simulink library "HILeg_Lib"  (R2014a)
settings: Solver=ode45  StartTime=0.0  StopTime=10.0  RelTol=1e-3
undefined symbols (not defined in the file): k_gx, k_gy, mu_slide, mu_stick, sgn, t_friction, v_gx_max, v_gy_max, vLimit
libraries: nesl_utility x7, simulink x5, sm_lib x3, simulink_extras x1
settings Model: Creator=rshum  LastModifiedBy=rshum

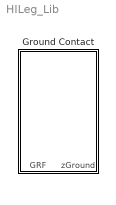
== system HILeg_Lib ==
  Ground Contact : Subsystem  SystemSampleTime=t_friction

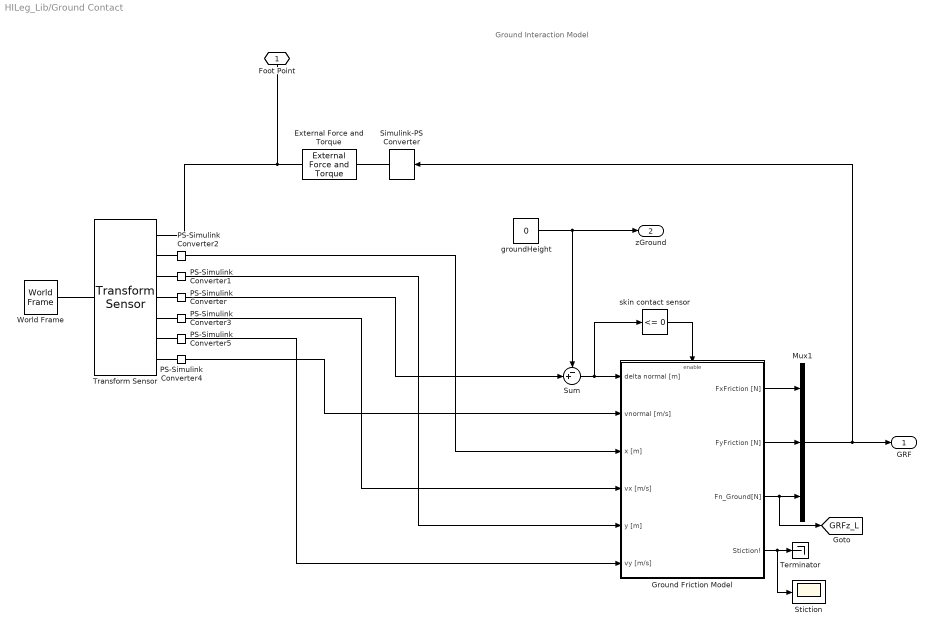
== system HILeg_Lib/Ground Contact ==
  note: Ground Interaction Model
  External Force and Torque : sm_lib/Forces and Torques/External Force and Torque  ForceResolutionFrame=World  EnableForceX=off  EnableForceY=off  EnableForceZ=off  EnableForce=on  TorqueResolutionFrame=AttachedFrame  EnableTorqueX=off  EnableTorqueY=off  EnableTorqueZ=off  EnableTorque=off  BlockFunction=simmechanics.library.forces_torques.external_force_torque
  Ground Friction Model : Subsystem
  Mux1 : Mux  Inputs=3
  PS-Simulink Converter{,1..5} (6 alike) : nesl_utility/PS-Simulink Converter  PhysicalDomain=network_engine_domain  SubClassName=ps_output  LeftPortType=input  RightPortType=output  PseudoPeriodic=off  Frequencies=[]  Unit=1  AffineConversion=off
  Simulink-PS Converter : nesl_utility/Simulink-PS Converter  PhysicalDomain=network_engine_domain  SubClassName=ps_input  LeftPortType=input  RightPortType=output  PseudoPeriodic=off  Frequencies=[]  NoiseDistribution=none  NoiseParameters=[]  Unit=1  AffineConversion=off  InputFiltering=off  SimscapeFilterOrder=1  InputFilterTimeConstant=0.001  UdotUserProvided=1
  Stiction : Scope
      settings: TimeRange=2.5  YMin=0  YMax=130  SaveName=ScopeData15
  Sum : Sum  Inputs=-+|
  Terminator : Terminator
  Transform Sensor : sm_lib/Frames and Transforms/Transform Sensor  MeasurementFrame=World  SenseAngle=off  SenseAxis=off  SenseAngle1=off  SenseAngle2=off  SenseAngle3=off  SenseQ=off  SenseR=off  SenseOmegaX=off  SenseOmegaY=off  SenseOmegaZ=off  SenseOmega1=off  SenseOmega2=off  SenseOmega3=off  SenseQDot=off  SenseRDot=off  SenseAlphaX=off  SenseAlphaY=off  SenseAlphaZ=off  SenseAlpha1=off  SenseAlpha2=off  SenseAlpha3=off  SenseQDDot=off  SenseRDDot=off  SenseX=on  SenseY=on  SenseZ=on  SenseRad=off  SenseAzim=off  SenseDist=off  SenseInc=off  SenseXDot=on  SenseYDot=on  SenseZDot=on  SenseRadDot=off  SenseAzimDot=off  SenseDistDot=off  SenseIncDot=off  SenseXDDot=off  SenseYDDot=off  SenseZDDot=off  SenseRadDDot=off  SenseAzimDDot=off  SenseDistDDot=off  SenseIncDDot=off  BlockFunction=simmechanics.library.frames_transforms.transform_sensor
  World Frame : sm_lib/Frames and Transforms/World Frame  BlockFunction=simmechanics.library.frames_transforms.world_frame
  groundHeight : Constant  Value=0
  skin contact sensor : simulink/Logic and Bit Operations/Compare To Zero  relop=<=  OutDataTypeStr=boolean
  Foot Point : PMIOPort  Port=1  Side=Left
  GRF : Outport
  zGround : Outport  Port=2
  tag scope: GRFz_L=global
  wires:
  Ground Friction Model/3(Fn_Ground[N]) -> Mux1/3, [GRFz_L]
  Ground Friction Model/2(FyFriction [N]) -> Mux1/2
  PS-Simulink Converter5/1 -> Ground Friction Model/6(vy [m/s])
  skin contact sensor/1 -> Ground Friction Model/Enable
  Mux1/1 -> GRF/1, Simulink-PS Converter/1
  groundHeight/1 -> Sum/1, zGround/1
  PS-Simulink Converter4/1 -> Ground Friction Model/2(vnormal [m/s])
  PS-Simulink Converter3/1 -> Ground Friction Model/4(vx [m/s])
  PS-Simulink Converter2/1 -> Ground Friction Model/3(x [m])
  PS-Simulink Converter1/1 -> Ground Friction Model/5(y [m])
  PS-Simulink Converter/1 -> Sum/2
  Ground Friction Model/4(Stiction!) -> Terminator/1, Stiction/1
  Ground Friction Model/1(FxFriction [N]) -> Mux1/1
  Sum/1 -> Ground Friction Model/1(delta normal [m]), skin contact sensor/1
  connections:
  World Frame/RConn1 -- Transform Sensor/LConn1
  Transform Sensor/RConn7 -- PS-Simulink Converter4/LConn1
  Transform Sensor/RConn6 -- PS-Simulink Converter5/LConn1
  PS-Simulink Converter3/LConn1 -- Transform Sensor/RConn5
  PS-Simulink Converter2/LConn1 -- Transform Sensor/RConn2
  Transform Sensor/RConn4 -- PS-Simulink Converter/LConn1
  Transform Sensor/RConn3 -- PS-Simulink Converter1/LConn1
  External Force and Torque/LConn1 -- Simulink-PS Converter/RConn1
  Foot Point/RConn1 -- Transform Sensor/RConn1 -- External Force and Torque/RConn1

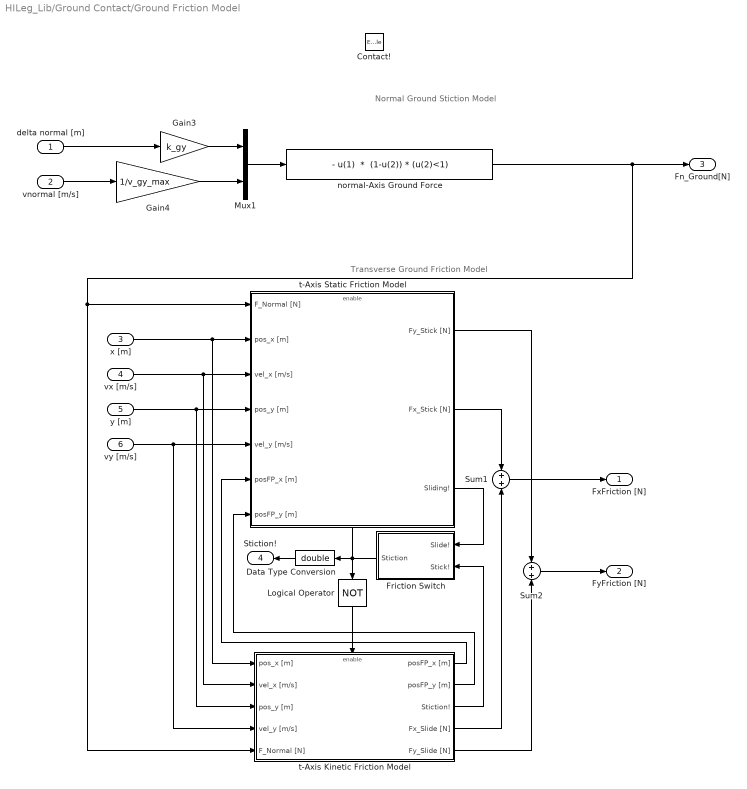
== system HILeg_Lib/Ground Contact/Ground Friction Model ==
  note: Normal Ground Stiction Model
  note: Transverse Ground Friction Model
  delta normal [m] : Inport
  vnormal [m/s] : Inport  Port=2
  x [m] : Inport  Port=3
  vx [m/s] : Inport  Port=4
  y [m] : Inport  Port=5
  vy [m/s] : Inport  Port=6
  Contact! : EnablePort  StatesWhenEnabling=reset
  Data Type Conversion : DataTypeConversion  OutDataTypeStr=double
  Friction Switch : Subsystem
  Gain3 : Gain  Gain=k_gy
  Gain4 : Gain  Gain=1/v_gy_max
  Logical Operator : Logic  Operator=NOT  AllPortsSameDT=off  OutDataTypeStr=boolean
  Mux1 : Mux  Inputs=2
  Sum1 : Sum
  Sum2 : Sum
  normal-Axis Ground Force : Fcn  Expr="- u(1)  *  (1-u(2)) * (u(2)<1)"
  t-Axis Kinetic Friction Model : Subsystem
  t-Axis Static Friction Model : Subsystem
  FxFriction [N] : Outport  OutputWhenDisabled=reset  InitialOutput=0
      settings: AttributesFormatString=initial = '%<InitialOutput>'\nwhen\ndisabled\n'%<OutputWhenDisabled>'
  FyFriction [N] : Outport  Port=2  OutputWhenDisabled=reset  InitialOutput=0
      settings: AttributesFormatString=initial = '%<InitialOutput>'\nwhen\ndisabled\n'%<OutputWhenDisabled>'
  Fn_Ground[N] : Outport  Port=3  OutputWhenDisabled=reset  InitialOutput=0
      settings: AttributesFormatString=initial = '%<InitialOutput>'\nwhen disabled = '%<OutputWhenDisabled>'
  Stiction! : Outport  Port=4  OutputWhenDisabled=reset  InitialOutput=0
      settings: AttributesFormatString=initial = '%<InitialOutput>'\nwhen\ndisabled\n'%<OutputWhenDisabled>'
  wires:
  Data Type Conversion/1 -> Stiction!/1
  vy [m/s]/1 -> t-Axis Static Friction Model/5(vel_y [m/s]), t-Axis Kinetic Friction Model/4(vel_y [m/s])
  y [m]/1 -> t-Axis Kinetic Friction Model/3(pos_y [m]), t-Axis Static Friction Model/4(pos_y [m])
  t-Axis Kinetic Friction Model/2(posFP_y [m]) -> t-Axis Static Friction Model/7(posFP_y [m])
  Sum2/1 -> FyFriction [N]/1
  t-Axis Kinetic Friction Model/5(Fy_Slide [N]) -> Sum2/2
  t-Axis Static Friction Model/1(Fy_Stick [N]) -> Sum2/1
  Gain4/1 -> Mux1/2
  Gain3/1 -> Mux1/1
  Mux1/1 -> normal-Axis Ground Force/1
  Logical Operator/1 -> t-Axis Kinetic Friction Model/Enable
  t-Axis Kinetic Friction Model/3(Stiction!) -> Friction Switch/2(Stick!)
  t-Axis Static Friction Model/3(Sliding!) -> Friction Switch/1(Slide!)
  Friction Switch/1(Stiction) -> t-Axis Static Friction Model/Enable, Logical Operator/1, Data Type Conversion/1
  Sum1/1 -> FxFriction [N]/1
  t-Axis Static Friction Model/2(Fx_Stick [N]) -> Sum1/1
  t-Axis Kinetic Friction Model/4(Fx_Slide [N]) -> Sum1/2
  t-Axis Kinetic Friction Model/1(posFP_x [m]) -> t-Axis Static Friction Model/6(posFP_x [m])
  vx [m/s]/1 -> t-Axis Static Friction Model/3(vel_x [m/s]), t-Axis Kinetic Friction Model/2(vel_x [m/s])
  x [m]/1 -> t-Axis Static Friction Model/2(pos_x [m]), t-Axis Kinetic Friction Model/1(pos_x [m])
  vnormal [m/s]/1 -> Gain4/1
  delta normal [m]/1 -> Gain3/1
  normal-Axis Ground Force/1 -> Fn_Ground[N]/1, t-Axis Kinetic Friction Model/5(F_Normal [N]), t-Axis Static Friction Model/1(F_Normal [N])

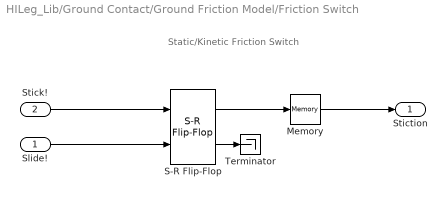
== system HILeg_Lib/Ground Contact/Ground Friction Model/Friction Switch ==
  note: Static/Kinetic Friction Switch
  Slide! : Inport
  Stick! : Inport  Port=2
  Memory : Memory  InheritSampleTime=on
  S-R Flip-Flop : simulink_extras/Flip Flops/S-R Flip-Flop  initial_condition=0
  Terminator : Terminator
  Stiction : Outport
  wires:
  Memory/1 -> Stiction/1
  Slide!/1 -> S-R Flip-Flop/2
  Stick!/1 -> S-R Flip-Flop/1
  S-R Flip-Flop/2 -> Terminator/1
  S-R Flip-Flop/1 -> Memory/1

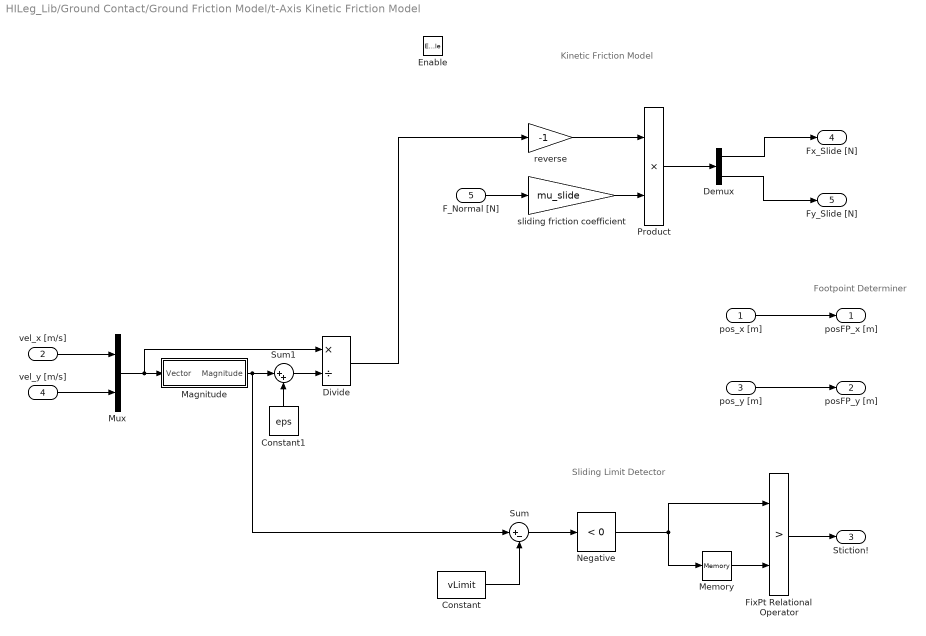
== system HILeg_Lib/Ground Contact/Ground Friction Model/t-Axis Kinetic Friction Model ==
  note: Sliding Limit Detector
  note: Footpoint Determiner
  note: Kinetic Friction Model
  pos_x [m] : Inport
  vel_x [m/s] : Inport  Port=2
  pos_y [m] : Inport  Port=3
  vel_y [m/s] : Inport  Port=4
  F_Normal [N] : Inport  Port=5
  Enable : EnablePort  StatesWhenEnabling=reset  ZeroCross=off
  Constant : Constant  Value=vLimit
  Constant1 : Constant  Value=eps
  Demux : Demux  Outputs=2
  Divide : Product  Inputs=*/
  FixPt Relational Operator : RelationalOperator  Operator=>  OutDataTypeStr=boolean  ZeroCross=off
  Magnitude : Subsystem
  Memory : Memory  InheritSampleTime=on
  Mux : Mux  Inputs=2
  Negative : simulink/Logic and Bit Operations/Compare To Zero  relop=<  OutDataTypeStr=boolean
  Product : Product  RndMeth=Zero
  Sum : Sum  Inputs=|+-
  Sum1 : Sum  Inputs=|++
  reverse : Gain  Gain=-1
  sliding friction coefficient : Gain  Gain=mu_slide
  posFP_x [m] : Outport  InitialOutput=0
      settings: AttributesFormatString=initial = '%<InitialOutput>'\nwhen disabled = '%<OutputWhenDisabled>'
  posFP_y [m] : Outport  Port=2  InitialOutput=0
      settings: AttributesFormatString=initial = '%<InitialOutput>'\nwhen disabled = '%<OutputWhenDisabled>'
  Stiction! : Outport  Port=3  OutputWhenDisabled=reset  InitialOutput=0
      settings: AttributesFormatString=initial = '%<InitialOutput>'\nwhen disabled = '%<OutputWhenDisabled>'
  Fx_Slide [N] : Outport  Port=4  OutputWhenDisabled=reset  InitialOutput=0
      settings: AttributesFormatString=initial = '%<InitialOutput>'\nwhen disabled = '%<OutputWhenDisabled>'
  Fy_Slide [N] : Outport  Port=5  OutputWhenDisabled=reset  InitialOutput=0
      settings: AttributesFormatString=initial = '%<InitialOutput>'\nwhen disabled = '%<OutputWhenDisabled>'
  wires:
  Demux/2 -> Fy_Slide [N]/1
  Demux/1 -> Fx_Slide [N]/1
  Product/1 -> Demux/1
  Sum1/1 -> Divide/2
  Constant1/1 -> Sum1/2
  Mux/1 -> Magnitude/1(Vector), Divide/1
  vel_y [m/s]/1 -> Mux/2
  vel_x [m/s]/1 -> Mux/1
  pos_y [m]/1 -> posFP_y [m]/1
  Constant/1 -> Sum/2
  Sum/1 -> Negative/1
  Magnitude/1(Magnitude) -> Sum1/1, Sum/1
  Negative/1 -> FixPt Relational Operator/1, Memory/1
  Memory/1 -> FixPt Relational Operator/2
  FixPt Relational Operator/1 -> Stiction!/1
  Divide/1 -> reverse/1
  sliding friction coefficient/1 -> Product/2
  pos_x [m]/1 -> posFP_x [m]/1
  F_Normal [N]/1 -> sliding friction coefficient/1
  reverse/1 -> Product/1

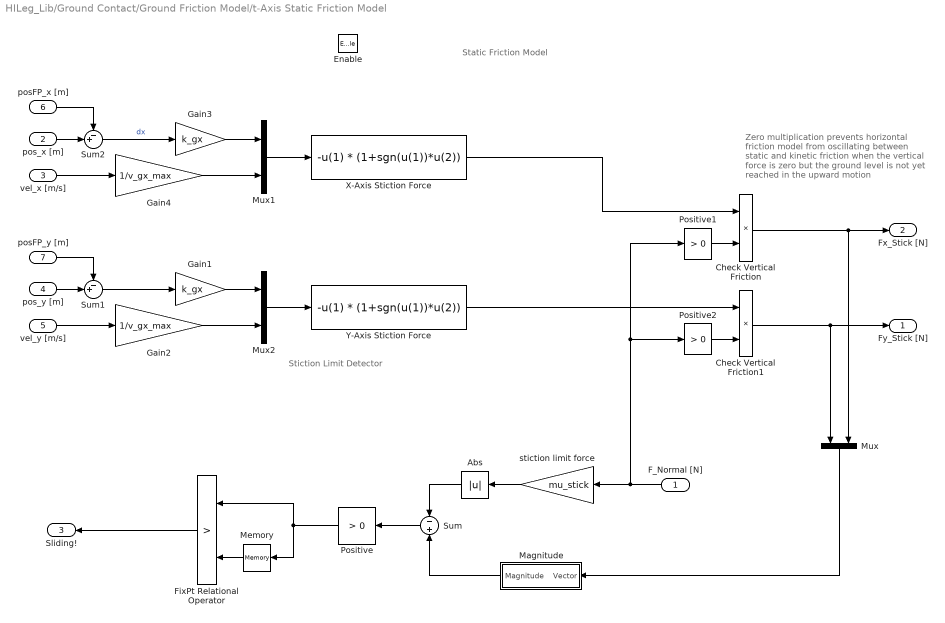
== system HILeg_Lib/Ground Contact/Ground Friction Model/t-Axis Static Friction Model ==
  note: Static Friction Model
  note: Stiction Limit Detector
  note: Zero multiplication prevents
      | horizontal friction model from
      | oscillating between static and kinetic
      | friction when the vertical force is zero but
      | the ground level is not yet reached
      | in the upward motion
  F_Normal [N] : Inport
  pos_x [m] : Inport  Port=2
  vel_x [m/s] : Inport  Port=3
  pos_y [m] : Inport  Port=4
  vel_y [m/s] : Inport  Port=5
  posFP_x [m] : Inport  Port=6
  posFP_y [m] : Inport  Port=7
  Enable : EnablePort  StatesWhenEnabling=reset  ZeroCross=off
  Abs : Abs
  Check Vertical Friction : Product  RndMeth=Zero
  Check Vertical Friction1 : Product  RndMeth=Zero
  FixPt Relational Operator : RelationalOperator  Operator=>  OutDataTypeStr=boolean  ZeroCross=off
  Gain1 : Gain  Gain=k_gx
  Gain2 : Gain  Gain=1/v_gx_max
  Gain3 : Gain  Gain=k_gx
  Gain4 : Gain  Gain=1/v_gx_max
  Magnitude : Subsystem
  Memory : Memory  InheritSampleTime=on
  Mux : Mux  Inputs=2
  Mux1 : Mux  Inputs=2
  Mux2 : Mux  Inputs=2
  Positive : simulink/Logic and Bit Operations/Compare To Zero  relop=>  OutDataTypeStr=boolean
  Positive1 : simulink/Logic and Bit Operations/Compare To Zero  relop=>  OutDataTypeStr=boolean
  Positive2 : simulink/Logic and Bit Operations/Compare To Zero  relop=>  OutDataTypeStr=boolean
  Sum : Sum  Inputs=-+
  Sum1 : Sum  Inputs=-+|
  Sum2 : Sum  Inputs=-+|
  X-Axis Stiction Force : Fcn  Expr=-u(1) * (1+sgn(u(1))*u(2))
  Y-Axis Stiction Force : Fcn  Expr=-u(1) * (1+sgn(u(1))*u(2))
  stiction limit force : Gain  Gain=mu_stick
  Fy_Stick [N] : Outport  OutputWhenDisabled=reset  InitialOutput=0
      settings: AttributesFormatString=when disabled: %<OutputWhenDisabled>\ninitial: %<InitialOutput>
  Fx_Stick [N] : Outport  Port=2  OutputWhenDisabled=reset  InitialOutput=0
      settings: AttributesFormatString=when disabled: %<OutputWhenDisabled>\ninitial: %<InitialOutput>
  Sliding! : Outport  Port=3  OutputWhenDisabled=reset  InitialOutput=0
      settings: AttributesFormatString=when disabled: %<OutputWhenDisabled>\ninitial: %<InitialOutput>
  wires:
  Sum1/1 -> Gain1/1
  Mux/1 -> Magnitude/1(Vector)
  Magnitude/1(Magnitude) -> Sum/2
  Check Vertical Friction1/1 -> Fy_Stick [N]/1, Mux/1
  Y-Axis Stiction Force/1 -> Check Vertical Friction1/1
  Positive2/1 -> Check Vertical Friction1/2
  pos_y [m]/1 -> Sum1/2
  posFP_y [m]/1 -> Sum1/1
  vel_y [m/s]/1 -> Gain2/1
  Mux2/1 -> Y-Axis Stiction Force/1
  Gain1/1 -> Mux2/1
  Gain2/1 -> Mux2/2
  F_Normal [N]/1 -> stiction limit force/1, Positive1/1, Positive2/1
  Sum2/1 -> Gain3/1  "dx"
  pos_x [m]/1 -> Sum2/2
  posFP_x [m]/1 -> Sum2/1
  vel_x [m/s]/1 -> Gain4/1
  Sum/1 -> Positive/1
  Memory/1 -> FixPt Relational Operator/2
  Positive/1 -> FixPt Relational Operator/1, Memory/1
  Mux1/1 -> X-Axis Stiction Force/1
  Gain3/1 -> Mux1/1
  Gain4/1 -> Mux1/2
  FixPt Relational Operator/1 -> Sliding!/1
  Abs/1 -> Sum/1
  stiction limit force/1 -> Abs/1
  X-Axis Stiction Force/1 -> Check Vertical Friction/1
  Positive1/1 -> Check Vertical Friction/2
  Check Vertical Friction/1 -> Fx_Stick [N]/1, Mux/2

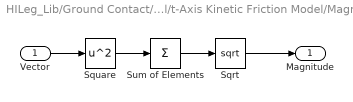
== system HILeg_Lib/Ground Contact/Ground Friction Model/t-Axis Kinetic Friction Model/Magnitude ==
  Vector : Inport
  Sqrt : Sqrt  OutputSignalType=real  SaturateOnIntegerOverflow=on
  Square : Math  Operator=square  OutputSignalType=real  SaturateOnIntegerOverflow=on
  Sum of Elements : Sum  Inputs=+
  Magnitude : Outport
  wires:
  Vector/1 -> Square/1
  Sum of Elements/1 -> Sqrt/1
  Square/1 -> Sum of Elements/1
  Sqrt/1 -> Magnitude/1

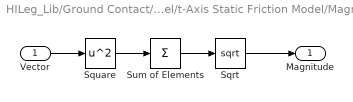
== system HILeg_Lib/Ground Contact/Ground Friction Model/t-Axis Static Friction Model/Magnitude ==
  Vector : Inport
  Sqrt : Sqrt  OutputSignalType=real  SaturateOnIntegerOverflow=on
  Square : Math  Operator=square  OutputSignalType=real  SaturateOnIntegerOverflow=on
  Sum of Elements : Sum  Inputs=+
  Magnitude : Outport
  wires:
  Vector/1 -> Square/1
  Sum of Elements/1 -> Sqrt/1
  Square/1 -> Sum of Elements/1
  Sqrt/1 -> Magnitude/1
